simulink model "FB_Controller_HIL"  (R2025b)
settings: Solver=FixedStepDiscrete  StartTime=0.0  StopTime=tspan  FixedStep=dt_sim  RelTol=rel_tol  AbsTol=abs_tol
undefined symbols (not defined in the file): const_voltage, mission_file
settings Model: Creator=koryh  LastModifiedBy=koryh

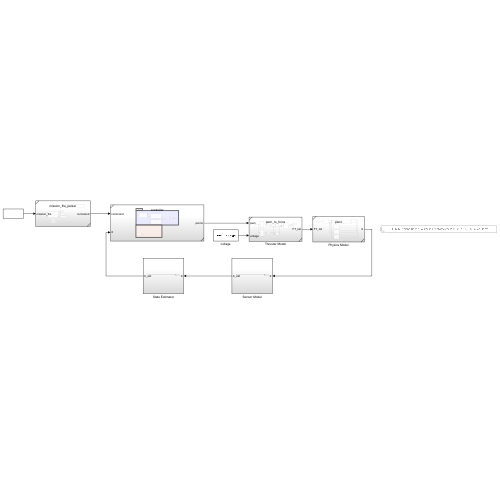
[thumbnail: Simulink's stored preview of the top-level diagram]
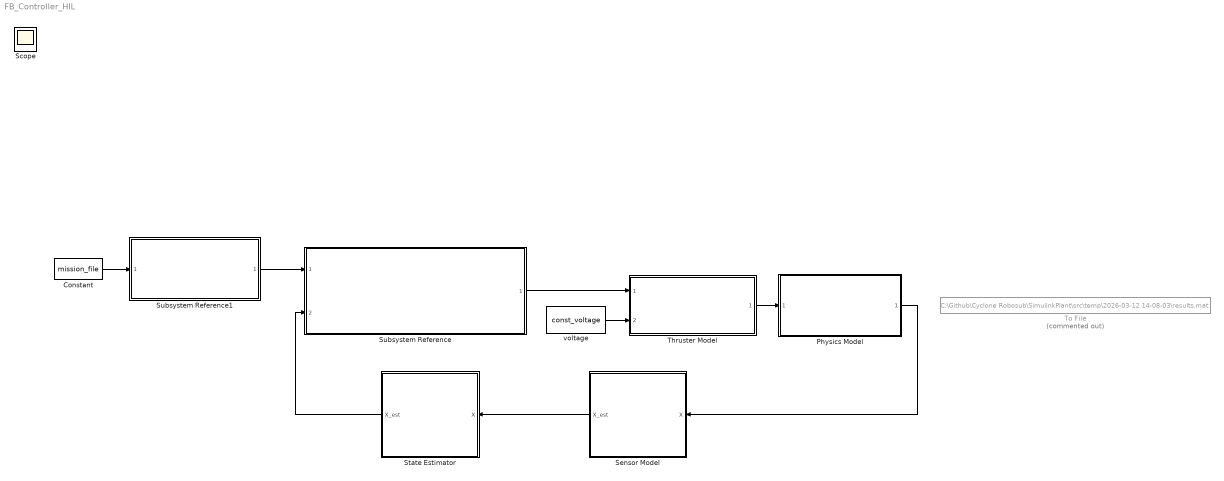
== system FB_Controller_HIL ==
  Constant : Constant  Value=mission_file
  Physics Model : Subsystem  ReferencedSubsystem=plant
  Sensor Model : Subsystem
  State Estimator : Subsystem
  Subsystem Reference : Subsystem  ReferencedSubsystem=controller
  Subsystem Reference1 : Subsystem  ReferencedSubsystem=mission_file_parser
  Thruster Model : Subsystem  ReferencedSubsystem=pwm_to_force
  To File : ToFile  Commented=on  Filename=C:\Github\Cyclone Robosub\SimulinkPlant\src\temp\2026-03-12 14-08-03\results.mat  MatrixName=X  SaveFormat=Timeseries
  voltage : Constant  Value=const_voltage
  Scope : Scope
      settings: ActiveDisplayYMinimum=-0.048832566475369238  ActiveDisplayYMaximum=0.79721663606048965
  wires:
  voltage/1 -> Thruster Model/2
  Subsystem Reference1/1 -> Subsystem Reference/1
  Constant/1 -> Subsystem Reference1/1
  State Estimator/1(X_est) -> Subsystem Reference/2
  Sensor Model/1(X_est) -> State Estimator/1(X)
  Subsystem Reference/1 -> Thruster Model/1
  Thruster Model/1 -> Physics Model/1
  Physics Model/1 -> Sensor Model/1(X)

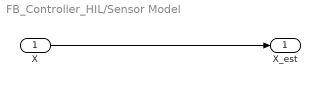
== system FB_Controller_HIL/Sensor Model ==
  X : Inport
  X_est : Outport
  wires:
  X/1 -> X_est/1

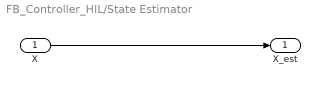
== system FB_Controller_HIL/State Estimator ==
  X : Inport
  X_est : Outport
  wires:
  X/1 -> X_est/1
